simulink model "HITL_DEMO"  (R2021b)
settings: Solver=FixedStepAuto  StartTime=0.0  StopTime=inf  FixedStep=.001  MaxStep=0.01  RelTol=1e-3
undefined symbols (not defined in the file or in its folder): Earth, WGS84
libraries: aerolibnav x2, etargetslib x2, mspfiltlib x1, aerolibutil x1, simulink x1, aerolibatmos2 x1, sharedtransform x1, aerolib6dof2 x1, instrumentlib x1
settings Model: Creator=kiran  LastModifiedBy=nikus
settings SolverCC: AutoInsertRateTranBlk=on

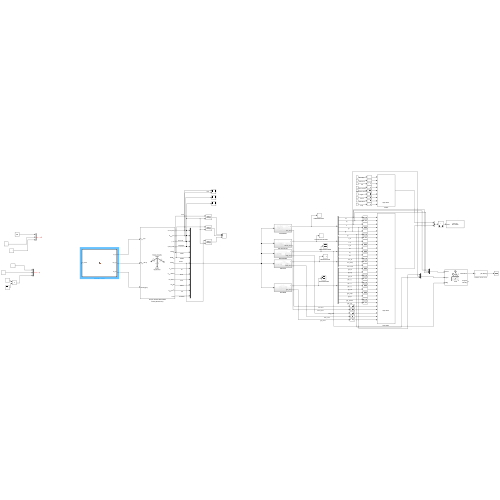
[thumbnail: Simulink's stored preview of the top-level diagram]
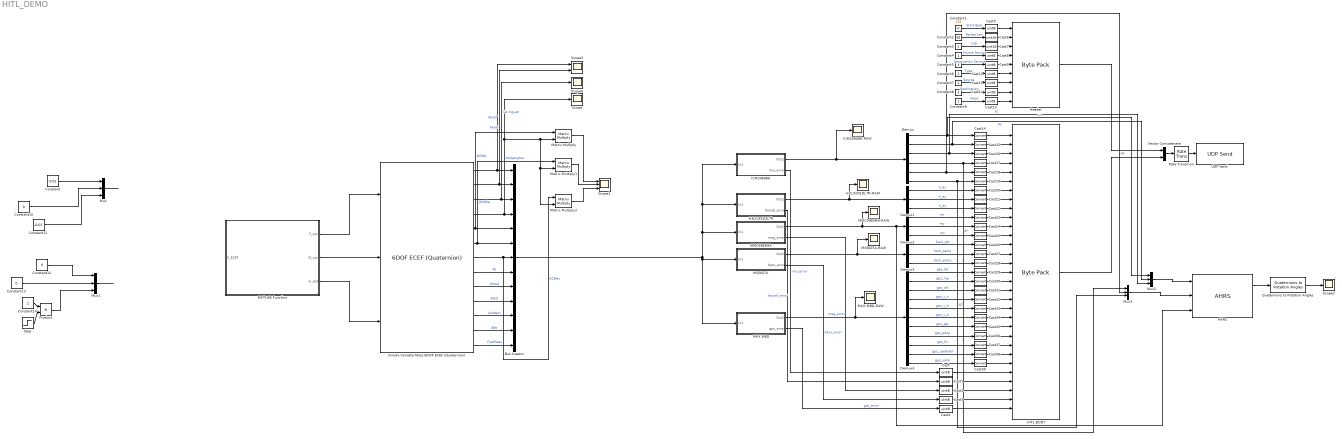
== system HITL_DEMO ==
  AHRS : mspfiltlib/AHRS  DispRefFrame=NED  DecimationFactor=1  InitialProcessNoise=ahrsfilter.defaultProcessNoise  OrientationFormat=quaternion  SimulateUsing=Interpreted execution  AccelerometerNoise=0.0001924722  GyroscopeNoise=9.1385e-5  MagnetometerNoise=0.1  GyroscopeDriftNoise=3.0462e-13  LinearAccelerationNoise=0.0096236100000000012  MagneticDisturbanceNoise=0.5  LinearAccelerationDecayFactor=0.5  MagneticDisturbanceDecayFactor=0.5  ExpectedMagneticFieldStrength=50
      settings: SourceProductBaseCode=TF,NV
  Bus Creator : BusCreator  Inputs=13
  Cast{,1..5,8..13} (12 alike) : DataTypeConversion  OutDataTypeStr=uint8
  Cast{14..39} (26 alike) : DataTypeConversion
  Cast6 : DataTypeConversion  OutDataTypeStr=uint16
  Cast7 : DataTypeConversion  OutDataTypeStr=uint16
  Constant : Constant  Value=0.01
  Constant1 : Constant  Value=175
  Constant10 : Constant  Value=0
  Constant11 : Constant  Value=-0.01
  Constant12 : Constant  Value=0
  Constant13 : Constant  Value=0
  Constant14 : Constant  Value=.1
  Constant2 : Constant  Value=95
  Constant{3..4,6..7,9} (5 alike) : Constant
  Constant5 : Constant  Value=3
  Constant8 : Constant  Value=2
  Demux : Demux  Outputs=6
  Demux1 : Demux  Outputs=3
  Demux2 : Demux  Outputs=3
  Demux3 : Demux  Outputs=3
  Demux4 : Demux  Outputs=11
  H3LIS331DLTR : Subsystem
  H3LIS331DLTR-RAW : Scope
  HITL BODY : etargetslib/Byte Pack  datatypes={'single','single','single','single','single','single','single','single','single','single','single','single','single','single','single','single','single','int32','int32','int32','int32','uint8','uint16','uint8','uint8','uint8','uint8','uint8','uint8','uint8','uint8'}  byteAlign=1
  Header : etargetslib/Byte Pack  datatypes={'uint8','uint16','uint16','uint8','uint8','uint8','uint8','uint8','uint8'}  byteAlign=1
  ICM20608G : Subsystem
  ICM20608G-RAW : Scope
  MATLAB Function : MATLAB Function  TreatAsAtomicUnit=on
  MAX M8Q : Subsystem
  MAX-M8Q-RAW : Scope
  MMC5983MA : Subsystem
  MMC5983MA-RAW : Scope
  MS5607A : Subsystem
  MS5607A-RAW : Scope
  Matrix Multiply : Product  Multiplication=Matrix(*)
  Matrix Multiply1 : Product  Multiplication=Matrix(*)
  Matrix Multiply2 : Product  Multiplication=Matrix(*)
  Mux{,1..3} (4 alike) : Mux  Inputs=3
  Product : Product
  Quaternions to Rotation Angles : sharedtransform/Quaternions to Rotation Angles  rotationOrder=ZYX  aMode=aMode
      settings: SourceProductBaseCode=AE,PW,DR,MT,UV,VE
  Rate Transition : RateTransition  OutPortSampleTime=.01
  Scope : Scope
  Scope1 : Scope  NumInputPorts=3
  Scope2 : Scope
  Scope5 : Scope  NumInputPorts=2
  Scope6 : Scope
  Simple Variable Mass 6DOF ECEF (Quaternion) : aerolib6dof2/6DOF ECEF (Quaternion)  units=Metric (MKS)  mtype=Simple Variable  xg_0=[0 0 0]  Vm_0=[0 0 0]  eul_0=[0 0 0]  pm_0=[0 0 0]  mass_0=1.0  mass_e=0.5  mass_f=2.0  inertia=eye(3)  inertia_e=eye(3)  inertia_f=2*eye(3)  vre_flag=off  abi_flag=off  ptype=Earth (WGS84)  R=6378137  F=1/298.257223563  w_E=7292115e-11  angle_in=Internal  LG0=0  quat_statename=''  pm_statename=''  Vm_statename=''  posECEF_statename=''  posECI_statename=''  LG_statename=''  mass_statename=''
      settings: SourceProductBaseCode=AE
  Step : Step  Time=10  Before=1  After=0  SampleTime=0
  UDP Send : instrumentlib/UDP Send  Host=127.0.0.1  Port=9090  LocalPort=-1  EnablePortSharing=off  ByteOrder=LittleEndian  OutputDatagramPacketSize=512  EnableBlockingMode=on  LocalAddress=0.0.0.0
  Vector Concatenate : Concatenate
  wires:
  Vector Concatenate/1 -> Rate Transition/1
  Header/1 -> Vector Concatenate/1
  HITL BODY/1 -> Vector Concatenate/2
  Demux/1 -> Mux2/1, Cast14/1  "ax"
  Demux/2 -> Mux2/2, Cast15/1  "ay"
  Demux/3 -> Mux2/3, Cast16/1  "az"
  Demux/4 -> Mux3/1, Cast17/1  "gx"
  Demux/6 -> Mux3/3, Cast19/1  "gz"
  Demux1/1 -> Cast20/1  "h_ax"
  Demux1/2 -> Cast21/1  "h_ay"
  Demux1/3 -> Cast22/1  "h_az"
  Demux2/1 -> Cast23/1  "mx"
  Demux2/2 -> Cast24/1  "my"
  Demux2/3 -> Cast25/1  "mz"
  Demux3/1 -> Cast26/1  "baro_alt"
  Demux3/2 -> Cast27/1  "baro_temp"
  Demux3/3 -> Cast28/1  "baro_press"
  Demux4/1 -> Cast29/1  "gps_lat"
  Demux4/2 -> Cast30/1  "gps_lng"
  Demux4/3 -> Cast31/1  "gps_alt"
  Demux4/4 -> Cast32/1  "gps_v_n"
  Demux4/5 -> Cast33/1  "gps_v_e"
  Demux4/6 -> Cast34/1  "gps_v_d"
  Demux4/7 -> Cast35/1  "gps_sat"
  Demux4/8 -> Cast36/1  "gps_pdop"
  Demux4/9 -> Cast37/1  "gps_fix"
  Demux4/10 -> Cast38/1  "gps_updated"
  Demux4/11 -> Cast39/1  "gps_valid"
  ICM20608G/2(imu_error) -> Cast/1  "imu_error"
  H3LIS331DLTR/2(haccel_error) -> Cast1/1  "haccel_error"
  MMC5983MA/2(mag_error) -> Cast2/1  "mag_error"
  MS5607A/2(baro_error) -> Cast3/1  "baro_error"
  MAX M8Q/2(gps_error) -> Cast4/1  "gps_error"
  Demux/5 -> Mux3/2, Cast18/1  "gy"
  ICM20608G/1(Out1) -> ICM20608G-RAW/1, Demux/1
  H3LIS331DLTR/1(Out1) -> H3LIS331DLTR-RAW/1, Demux1/1
  MMC5983MA/1(Out1) -> MMC5983MA-RAW/1, AHRS/3, Demux2/1
  MS5607A/1(Out1) -> MS5607A-RAW/1, Demux3/1
  MAX M8Q/1(Out1) -> MAX-M8Q-RAW/1, Demux4/1
  Constant1/1 -> Cast5/1  "Start Byte"
  Constant2/1 -> Cast6/1  "Packet Len"
  Constant3/1 -> Cast7/1  "UID"
  Constant4/1 -> Cast8/1  "Source Service"
  Constant5/1 -> Cast9/1  "Destination Service"
  Constant6/1 -> Cast10/1  "Type"
  Constant7/1 -> Cast11/1  "Source"
  Constant8/1 -> Cast12/1  "Destination"
  Constant9/1 -> Cast13/1  "Hops"
  Simple Variable Mass 6DOF ECEF (Quaternion)/2 -> Scope5/2, Bus Creator/2  "Xecef"
  Simple Variable Mass 6DOF ECEF (Quaternion)/3 -> Scope6/1, Bus Creator/3  "lat,lng,alt"
  Simple Variable Mass 6DOF ECEF (Quaternion)/4 -> Matrix Multiply2/2, Matrix Multiply1/2, Matrix Multiply/2, Scope/1, Bus Creator/4  "bodyangles"
  Simple Variable Mass 6DOF ECEF (Quaternion)/8 -> Bus Creator/8  "Vb"
  Simple Variable Mass 6DOF ECEF (Quaternion)/9 -> Bus Creator/9  "Wned"
  Simple Variable Mass 6DOF ECEF (Quaternion)/10 -> Bus Creator/10  "Wecl"
  Simple Variable Mass 6DOF ECEF (Quaternion)/11 -> Bus Creator/11  "dwdtecl"
  Simple Variable Mass 6DOF ECEF (Quaternion)/12 -> Bus Creator/12  "Abb"
  Simple Variable Mass 6DOF ECEF (Quaternion)/5 -> Bus Creator/5, Matrix Multiply/1  "DCMbi"
  Simple Variable Mass 6DOF ECEF (Quaternion)/6 -> Bus Creator/6, Matrix Multiply1/1  "DCMbe"
  Simple Variable Mass 6DOF ECEF (Quaternion)/7 -> Matrix Multiply2/1, Bus Creator/7  "DCMec"
  Mux/1 -> ?
  Constant/1 -> Mux/1
  Constant10/1 -> Mux/2
  Constant11/1 -> Mux/3
  Product/1 -> Mux1/3
  Constant12/1 -> Mux1/1
  Constant13/1 -> Mux1/2
  Mux1/1 -> ?
  Cast2/1 -> HITL BODY/29
  Cast3/1 -> HITL BODY/30
  Cast4/1 -> HITL BODY/31
  Cast5/1 -> Header/1
  Cast6/1 -> Header/2
  Cast7/1 -> Header/3
  Cast8/1 -> Header/4
  Cast9/1 -> Header/5
  Cast10/1 -> Header/6
  Cast11/1 -> Header/7
  Cast12/1 -> Header/8
  Cast13/1 -> Header/9
  Cast14/1 -> HITL BODY/1
  Cast15/1 -> HITL BODY/2
  Cast16/1 -> HITL BODY/3
  Cast17/1 -> HITL BODY/4
  Cast18/1 -> HITL BODY/5
  Cast19/1 -> HITL BODY/6
  Cast20/1 -> HITL BODY/7
  Cast25/1 -> HITL BODY/12
  Cast23/1 -> HITL BODY/10
  Cast27/1 -> HITL BODY/14
  Cast26/1 -> HITL BODY/13
  Cast22/1 -> HITL BODY/9
  Cast24/1 -> HITL BODY/11
  Cast21/1 -> HITL BODY/8
  Cast39/1 -> HITL BODY/26
  Cast/1 -> HITL BODY/27
  Cast1/1 -> HITL BODY/28
  Cast36/1 -> HITL BODY/23
  Cast38/1 -> HITL BODY/25
  Cast37/1 -> HITL BODY/24
  Cast35/1 -> HITL BODY/22
  Cast33/1 -> HITL BODY/20
  Cast32/1 -> HITL BODY/19
  Cast34/1 -> HITL BODY/21
  Cast31/1 -> HITL BODY/18
  Cast28/1 -> HITL BODY/15
  Cast30/1 -> HITL BODY/17
  Cast29/1 -> HITL BODY/16
  Bus Creator/1 -> MMC5983MA/1(In1), ICM20608G/1(In1), H3LIS331DLTR/1(In1), MAX M8Q/1(In1), MS5607A/1(In1)
  Simple Variable Mass 6DOF ECEF (Quaternion)/1 -> Scope5/1, Bus Creator/1  "Vecef"
  Rate Transition/1 -> UDP Send/1
  Constant14/1 -> Product/1
  Step/1 -> Product/2
  Matrix Multiply/1 -> Scope1/1
  Matrix Multiply1/1 -> Scope1/2
  Matrix Multiply2/1 -> Scope1/3
  Mux2/1 -> AHRS/1
  Mux3/1 -> AHRS/2
  AHRS/1 -> Quaternions to Rotation Angles/1
  Quaternions to Rotation Angles/1 -> Scope2/1
  Simple Variable Mass 6DOF ECEF (Quaternion)/13 -> Bus Creator/13  "FuelMass"
  MATLAB Function/1(F_xyz) -> Simple Variable Mass 6DOF ECEF (Quaternion)/1
  MATLAB Function/2(M_xyz) -> Simple Variable Mass 6DOF ECEF (Quaternion)/2
  MATLAB Function/3(m_dot) -> Simple Variable Mass 6DOF ECEF (Quaternion)/3

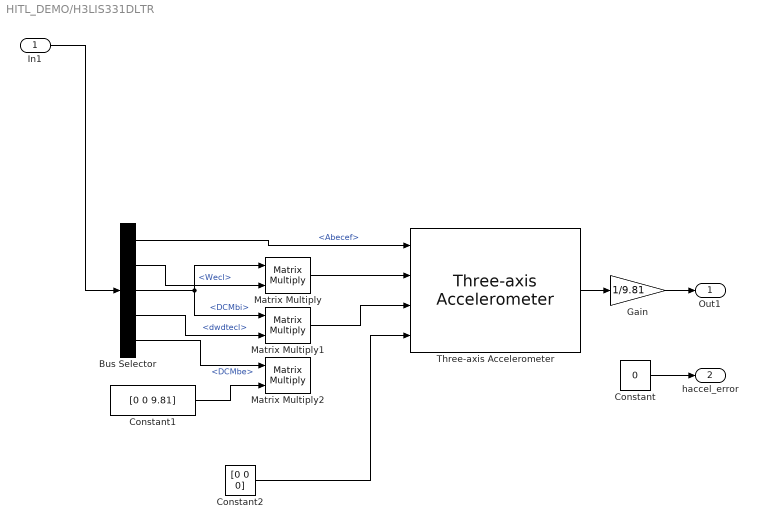
== system HITL_DEMO/H3LIS331DLTR ==
  In1 : Inport
  Bus Selector : BusSelector  OutputSignals=Abecef,Wecl,DCMbi,dwdtecl,DCMbe
  Constant : Constant  Value=0
  Constant1 : Constant  Value=[0 0 9.81]
  Constant2 : Constant  Value=[0 0 0]
  Gain : Gain  Gain=1/9.81
  Matrix Multiply : Product  Multiplication=Matrix(*)
  Matrix Multiply1 : Product  Multiplication=Matrix(*)
  Matrix Multiply2 : Product  Multiplication=Matrix(*)
  Three-axis Accelerometer : aerolibnav/Three-axis Accelerometer  units=Metric (MKS)  acc=[0 0 0]  gtype=off  dtype_a=on  w_a=190  z_a=0.707  a_sf_cc=[1 0 0; 0 1 0; 0 0 1]  a_bias=[0 0 0]  a_Ts=0  a_rand=off  a_seeds=[23093 23094 23095]  a_pow=[0.001 0.001 0.001]  a_sat="[-inf  -inf  -inf  inf inf inf]"
      settings: SourceProductBaseCode=AE
  Out1 : Outport
  haccel_error : Outport  Port=2
  wires:
  In1/1 -> Bus Selector/1
  Bus Selector/5 -> Matrix Multiply2/1  "<DCMbe>"
  Bus Selector/2 -> Matrix Multiply/2  "<Wecl>"
  Constant2/1 -> Three-axis Accelerometer/4
  Bus Selector/3 -> Matrix Multiply1/1, Matrix Multiply/1  "<DCMbi>"
  Matrix Multiply1/1 -> Three-axis Accelerometer/3
  Constant1/1 -> Matrix Multiply2/2
  Bus Selector/4 -> Matrix Multiply1/2  "<dwdtecl>"
  Matrix Multiply/1 -> Three-axis Accelerometer/2
  Bus Selector/1 -> Three-axis Accelerometer/1  "<Abecef>"
  Constant/1 -> haccel_error/1
  Three-axis Accelerometer/1 -> Gain/1
  Gain/1 -> Out1/1

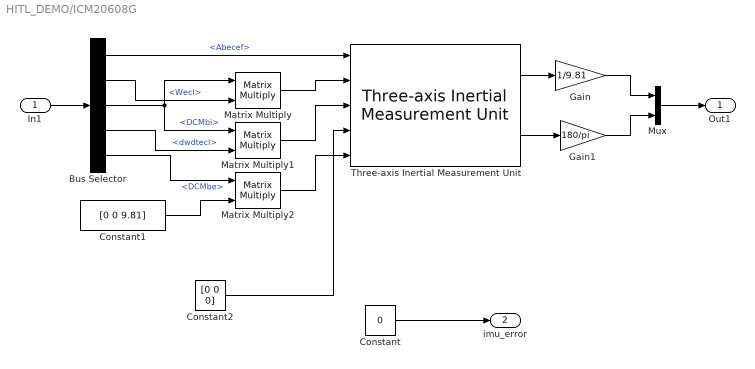
== system HITL_DEMO/ICM20608G ==
  In1 : Inport
  Bus Selector : BusSelector  OutputSignals=Abecef,Wecl,DCMbi,dwdtecl,DCMbe
  Constant : Constant  Value=0
  Constant1 : Constant  Value=[0 0 9.81]
  Constant2 : Constant  Value=[0 0 0]
  Gain : Gain  Gain=1/9.81
  Gain1 : Gain  Gain=180/pi
  Matrix Multiply : Product  Multiplication=Matrix(*)
  Matrix Multiply1 : Product  Multiplication=Matrix(*)
  Matrix Multiply2 : Product  Multiplication=Matrix(*)
  Mux : Mux  Inputs=2
  Three-axis Inertial Measurement Unit : aerolibnav/Three-axis Inertial Measurement Unit  units=Metric (MKS)  imu=[0 0 0]  i_Ts=0.01  dtype_a=on  w_a=190  z_a=0.707  a_sf_cc=[1 0 0; 0 1 0; 0 0 1]  a_bias=[0 0 0]  a_sat="[-16  -16  -16  16 16 16]*9.81"  dtype_g=on  w_g=190  z_g=0.707  g_sf_cc=[1 0 0; 0 1 0; 0 0 1]  g_bias=[0 0 0]  g_sens=[0 0 0]  g_sat="[-inf  -inf  -inf  inf inf inf]"  i_rand=off  i_seeds=[23093 23094 23095 23096 23097 23098]  i_pow=[0.001 0.001 0.001 0.0001 0.0001 0.0001]
  Out1 : Outport
  imu_error : Outport  Port=2
  wires:
  Constant/1 -> imu_error/1
  In1/1 -> Bus Selector/1
  Bus Selector/1 -> Three-axis Inertial Measurement Unit/1  "<Abecef>"
  Bus Selector/3 -> Matrix Multiply1/1, Matrix Multiply/1  "<DCMbi>"
  Bus Selector/4 -> Matrix Multiply1/2  "<dwdtecl>"
  Bus Selector/5 -> Matrix Multiply2/1  "<DCMbe>"
  Matrix Multiply/1 -> Three-axis Inertial Measurement Unit/2
  Bus Selector/2 -> Matrix Multiply/2  "<Wecl>"
  Matrix Multiply1/1 -> Three-axis Inertial Measurement Unit/3
  Constant1/1 -> Matrix Multiply2/2
  Matrix Multiply2/1 -> Three-axis Inertial Measurement Unit/5
  Constant2/1 -> Three-axis Inertial Measurement Unit/4
  Three-axis Inertial Measurement Unit/1 -> Gain/1
  Three-axis Inertial Measurement Unit/2 -> Gain1/1
  Mux/1 -> Out1/1
  Gain/1 -> Mux/1
  Gain1/1 -> Mux/2

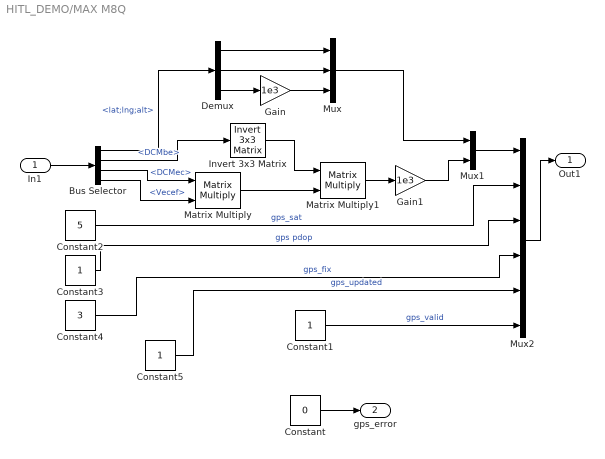
== system HITL_DEMO/MAX M8Q ==
  In1 : Inport
  Bus Selector : BusSelector  OutputSignals=lat;lng;alt,DCMbe,DCMec,Vecef
  Constant : Constant  Value=0
  Constant1 : Constant
  Constant2 : Constant  Value=5
  Constant3 : Constant
  Constant4 : Constant  Value=3
  Constant5 : Constant
  Demux : Demux  Outputs=3
  Gain : Gain  Gain=1e3
  Gain1 : Gain  Gain=1e3
  Invert 3x3 Matrix : aerolibutil/Invert  3x3 Matrix
  Matrix Multiply : Product  Multiplication=Matrix(*)
  Matrix Multiply1 : Product  Multiplication=Matrix(*)
  Mux : Mux  Inputs=3
  Mux1 : Mux  Inputs=2
  Mux2 : Mux  Inputs=6
  Out1 : Outport
  gps_error : Outport  Port=2
  wires:
  In1/1 -> Bus Selector/1
  Bus Selector/4 -> Matrix Multiply/2  "<Vecef>"
  Bus Selector/3 -> Matrix Multiply/1  "<DCMec>"
  Bus Selector/2 -> Invert 3x3 Matrix/1  "<DCMbe>"
  Bus Selector/1 -> Demux/1  "<lat;lng;alt>"
  Demux/1 -> Mux/1
  Demux/2 -> Mux/2
  Demux/3 -> Gain/1
  Gain/1 -> Mux/3
  Mux/1 -> Mux1/1
  Invert 3x3 Matrix/1 -> Matrix Multiply1/1
  Matrix Multiply/1 -> Matrix Multiply1/2
  Matrix Multiply1/1 -> Gain1/1
  Mux1/1 -> Mux2/1
  Gain1/1 -> Mux1/2
  Constant/1 -> gps_error/1
  Mux2/1 -> Out1/1
  Constant2/1 -> Mux2/2  "gps_sat"
  Constant3/1 -> Mux2/3  "gps pdop"
  Constant4/1 -> Mux2/4  "gps_fix"
  Constant5/1 -> Mux2/5  "gps_updated"
  Constant1/1 -> Mux2/6  "gps_valid"

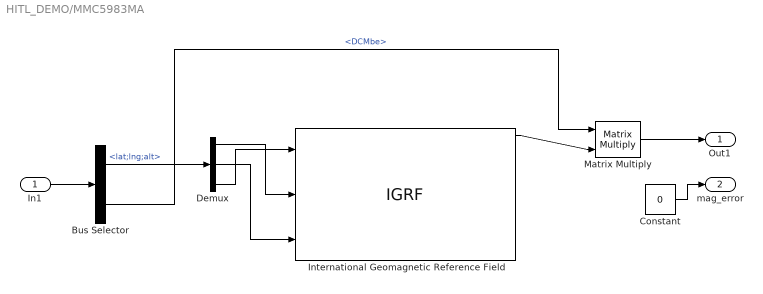
== system HITL_DEMO/MMC5983MA ==
  In1 : Inport
  Bus Selector : BusSelector  OutputSignals=lat;lng;alt,DCMbe
  Constant : Constant  Value=0
  Demux : Demux  Outputs=3
  International Geomagnetic Reference Field : IGRF  time_in=off  month=January  day=1  year=2020
      settings: AttributesFormatString=%<generation>
  Matrix Multiply : Product  Multiplication=Matrix(*)
  Out1 : Outport
  mag_error : Outport  Port=2
  wires:
  In1/1 -> Bus Selector/1
  Bus Selector/1 -> Demux/1  "<lat;lng;alt>"
  Demux/1 -> International Geomagnetic Reference Field/2
  Demux/2 -> International Geomagnetic Reference Field/3
  Demux/3 -> International Geomagnetic Reference Field/1
  Bus Selector/2 -> Matrix Multiply/1  "<DCMbe>"
  International Geomagnetic Reference Field/1 -> Matrix Multiply/2
  Matrix Multiply/1 -> Out1/1
  Constant/1 -> mag_error/1

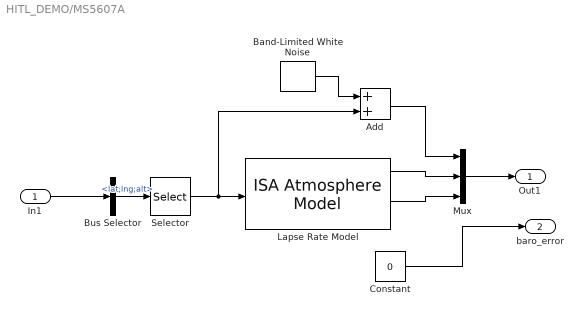
== system HITL_DEMO/MS5607A ==
  In1 : Inport
  Add : Sum
  Band-Limited White Noise : simulink/Sources/Band-Limited White Noise  Cov=[0.001]  Ts=0.01  seed=[23341]
  Bus Selector : BusSelector  OutputSignals=lat;lng;alt
  Constant : Constant  Value=0
  Lapse Rate Model : aerolibatmos2/ISA Atmosphere Model  custom=on  g=9.80665  gamma=1.4  R=287.0531  L=0.0065  h_trop=11000  h_strat=20000  rho0=1.225  P0=101325  T0=288.15  h0=0
  Mux : Mux  Inputs=3
  Selector : Selector  InputPortWidth=3  IndexOptions=Index vector (dialog)  Indices=3  OutputSizes=1
  Out1 : Outport
  baro_error : Outport  Port=2
  wires:
  In1/1 -> Bus Selector/1
  Bus Selector/1 -> Selector/1  "<lat;lng;alt>"
  Selector/1 -> Add/2, Lapse Rate Model/1
  Band-Limited White Noise/1 -> Add/1
  Add/1 -> Mux/1
  Lapse Rate Model/3 -> Mux/3
  Lapse Rate Model/1 -> Mux/2
  Mux/1 -> Out1/1
  Constant/1 -> baro_error/1

== matlab function HITL_DEMO/MATLAB Function ==
  data: V_ECEF input; F_xyz output; M_xyz output; m_dot output
function [F_xyz, M_xyz, m_dot] = fcn(V_ECEF)

y = u;
